simulink model "ModeloMotorDC"  (R2016a)
settings: Solver=VariableStepAuto  StartTime=0.0  StopTime=0.2  RelTol=1e-3
libraries: simulink x2, powerlib_meascontrol x2
settings Model: Creator=Juan  LastModifiedBy=Juan

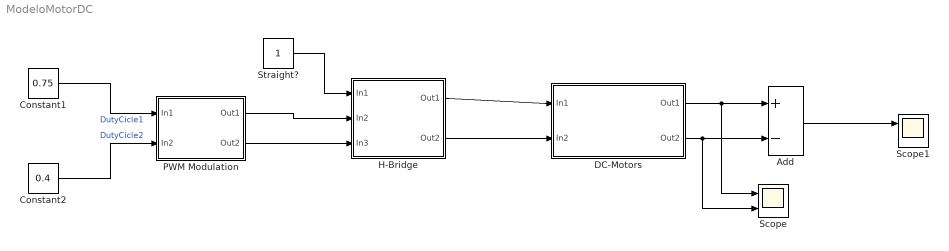
== system ModeloMotorDC ==
  Add : Sum  Inputs=+-
  Constant1 : Constant  Value=0.75
  Constant2 : Constant  Value=0.4
  "DC-Motors " : Subsystem
  "H-Bridge " : Subsystem
  PWM Modulation : Subsystem
  Scope : Scope  NumInputPorts=2
  Scope1 : Scope  NumInputPorts=2
  Straight? : Constant
  wires:
  Straight?/1 -> "H-Bridge "/1(In1)
  PWM Modulation/1(Out1) -> "H-Bridge "/2(In2)
  PWM Modulation/2(Out2) -> "H-Bridge "/3(In3)
  Constant1/1 -> PWM Modulation/1(In1)  "DutyCicle1"
  Constant2/1 -> PWM Modulation/2(In2)  "DutyCicle2"
  "H-Bridge "/1(Out1) -> "DC-Motors "/1(In1)
  "H-Bridge "/2(Out2) -> "DC-Motors "/2(In2)
  "DC-Motors "/1(Out1) -> Scope/1, Add/1
  "DC-Motors "/2(Out2) -> Add/2, Scope/2
  Add/1 -> Scope1/1

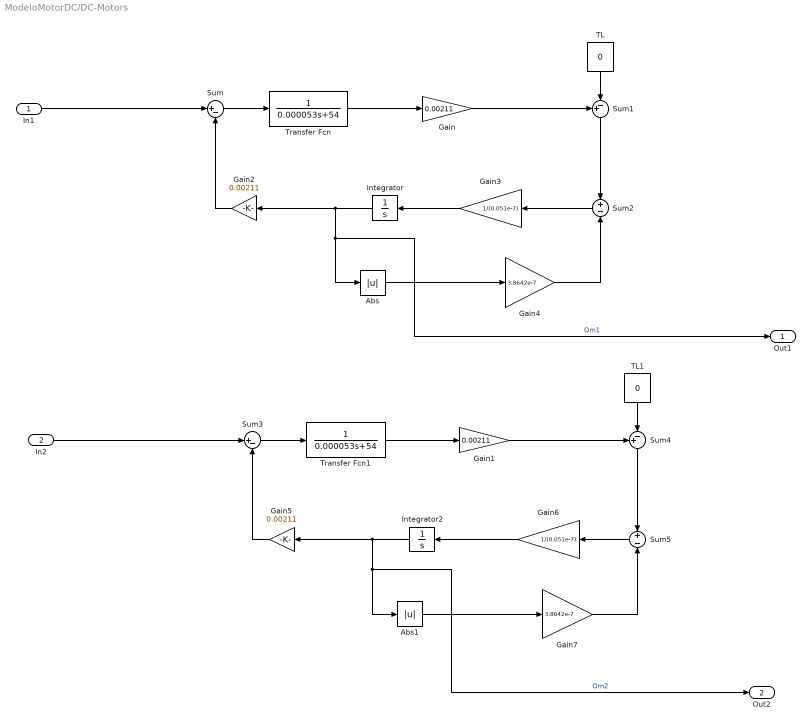
== system ModeloMotorDC/DC-Motors  ==
  In1 : Inport
  In2 : Inport  Port=2
  Abs : Abs
  Abs1 : Abs
  Gain{,1..2,5} (4 alike) : Gain  Gain=0.00211
  Gain3 : Gain  Gain=1/(0.051e-7)
  Gain4 : Gain  Gain=3.8642e-7
  Gain6 : Gain  Gain=1/(0.051e-7)
  Gain7 : Gain  Gain=3.8642e-7
  Integrator : Integrator
  Integrator2 : Integrator
  Sum : Sum  Inputs=|+-
  Sum1 : Sum  Inputs=+-|
  Sum2 : Sum  Inputs=+|-
  Sum3 : Sum  Inputs=|+-
  Sum4 : Sum  Inputs=+-|
  Sum5 : Sum  Inputs=+|-
  TL : Constant  Value=0
  TL1 : Constant  Value=0
  Transfer Fcn : TransferFcn  Denominator=[0.000053 54]
  Transfer Fcn1 : TransferFcn  Denominator=[0.000053 54]
  Out1 : Outport
  Out2 : Outport  Port=2
  wires:
  TL1/1 -> Sum4/2
  In2/1 -> Sum3/1
  Transfer Fcn1/1 -> Gain1/1
  Sum3/1 -> Transfer Fcn1/1
  Sum4/1 -> Sum5/1
  Gain6/1 -> Integrator2/1
  Integrator2/1 -> Gain5/1, Out2/1, Abs1/1  "Om2"
  Gain1/1 -> Sum4/1
  Gain5/1 -> Sum3/2
  Gain7/1 -> Sum5/2
  Abs1/1 -> Gain7/1
  Sum5/1 -> Gain6/1
  Sum/1 -> Transfer Fcn/1
  Gain/1 -> Sum1/1
  Transfer Fcn/1 -> Gain/1
  In1/1 -> Sum/1
  Integrator/1 -> Gain2/1, Out1/1, Abs/1  "Om1"
  Gain2/1 -> Sum/2
  Gain4/1 -> Sum2/2
  Sum1/1 -> Sum2/1
  Abs/1 -> Gain4/1
  Gain3/1 -> Integrator/1
  TL/1 -> Sum1/2
  Sum2/1 -> Gain3/1

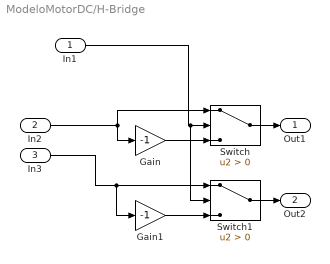
== system ModeloMotorDC/H-Bridge  ==
  In1 : Inport
  In2 : Inport  Port=2
  In3 : Inport  Port=3
  Gain : Gain  Gain=-1
  Gain1 : Gain  Gain=-1
  Switch : Switch  Criteria=u2 > Threshold
  Switch1 : Switch  Criteria=u2 > Threshold
  Out1 : Outport
  Out2 : Outport  Port=2
  wires:
  Switch/1 -> Out1/1
  Switch1/1 -> Out2/1
  Gain/1 -> Switch/3
  In2/1 -> Switch/1, Gain/1
  Gain1/1 -> Switch1/3
  In3/1 -> Gain1/1, Switch1/1
  In1/1 -> Switch1/2, Switch/2

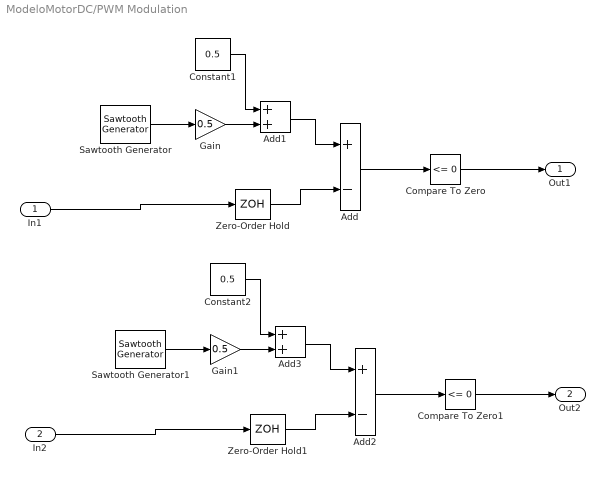
== system ModeloMotorDC/PWM Modulation ==
  In1 : Inport
  In2 : Inport  Port=2
  Add : Sum  Inputs=+-
  Add1 : Sum
  Add2 : Sum  Inputs=+-
  Add3 : Sum
  Compare To Zero : simulink/Logic and Bit Operations/Compare To Zero  relop=<=  OutDataTypeStr=boolean
  Compare To Zero1 : simulink/Logic and Bit Operations/Compare To Zero  relop=<=  OutDataTypeStr=boolean
  Constant1 : Constant  Value=0.5
  Constant2 : Constant  Value=0.5
  Gain : Gain  Gain=0.5
  Gain1 : Gain  Gain=0.5
  Sawtooth Generator : powerlib_meascontrol/Pulse & Signal Generators/Sawtooth Generator  Freq=500  Phase=0  Ts=0
  Sawtooth Generator1 : powerlib_meascontrol/Pulse & Signal Generators/Sawtooth Generator  Freq=500  Phase=0  Ts=0
  Zero-Order Hold : ZeroOrderHold  SampleTime=-1
  Zero-Order Hold1 : ZeroOrderHold  SampleTime=-1
  Out1 : Outport
  Out2 : Outport  Port=2
  wires:
  Zero-Order Hold/1 -> Add/2
  Compare To Zero/1 -> Out1/1
  Add1/1 -> Add/1
  Constant1/1 -> Add1/1
  Gain/1 -> Add1/2
  Sawtooth Generator/1 -> Gain/1
  In2/1 -> Zero-Order Hold1/1
  Add3/1 -> Add2/1
  Gain1/1 -> Add3/2
  Sawtooth Generator1/1 -> Gain1/1
  Constant2/1 -> Add3/1
  Add2/1 -> Compare To Zero1/1
  Zero-Order Hold1/1 -> Add2/2
  Compare To Zero1/1 -> Out2/1
  In1/1 -> Zero-Order Hold/1
  Add/1 -> Compare To Zero/1
